simulink model "problem_2"  (R2020b)
settings: Solver=VariableStepAuto  StartTime=0.0  StopTime=10.0  RelTol=1e-3
settings Model: Creator=hp  LastModifiedBy=hp

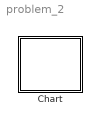
== system problem_2 ==
  Chart : Stateflow chart  TreatAsAtomicUnit=on

== stateflow chart problem_2/Chart ==
  settings: stateMachineType=MOORE_MACHINE
